simulink model "WhileIteratorSubsystem"  (R2015b)
settings: Solver=VariableStepAuto  StartTime=0.0  StopTime=10.0  RelTol=1e-3
settings Model: Creator=LUBO  LastModifiedBy=LUBO

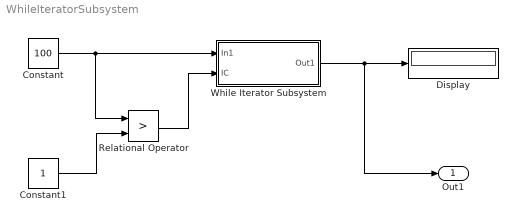
== system WhileIteratorSubsystem ==
  Constant : Constant  Value=100
  Constant1 : Constant
  Display : Display
  Relational Operator : RelationalOperator  Operator=>  OutDataTypeStr=boolean
  While Iterator Subsystem : Subsystem  TreatAsAtomicUnit=on
  Out1 : Outport
  wires:
  Constant/1 -> Relational Operator/1, While Iterator Subsystem/1(In1)
  Constant1/1 -> Relational Operator/2
  Relational Operator/1 -> While Iterator Subsystem/2(IC)
  While Iterator Subsystem/1(Out1) -> Out1/1, Display/1

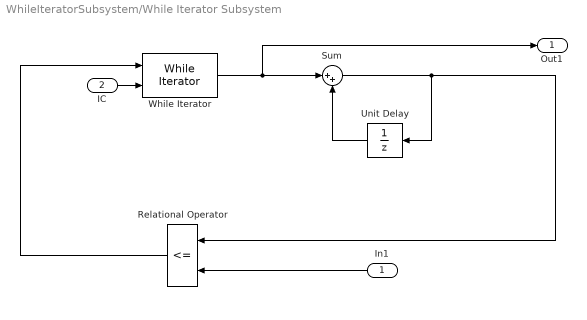
== system WhileIteratorSubsystem/While Iterator Subsystem ==
  In1 : Inport
  IC : Inport  Port=2
  Relational Operator : RelationalOperator  Operator=<=  OutDataTypeStr=boolean
  Sum : Sum  Inputs=|++
  Unit Delay : UnitDelay  SampleTime=-1
  While Iterator : WhileIterator  MaxIters=1000  ResetStates=reset  ShowIterationPort=on  OutputDataType=double
  Out1 : Outport
  wires:
  IC/1 -> While Iterator/2
  In1/1 -> Relational Operator/2
  Relational Operator/1 -> While Iterator/1
  While Iterator/1 -> Out1/1, Sum/1
  Sum/1 -> Unit Delay/1, Relational Operator/1
  Unit Delay/1 -> Sum/2
